simulink model "SIM_SAD_DEMO"  (R2025b)
settings: Solver=ode5  StartTime=0.0  StopTime=T/10  FixedStep=0.1  RelTol=1e-3
model workspace (MAT data in the model file):
  Pnull : Simulink.Parameter (value not decoded)
  rho_albedo_medio : Simulink.Parameter (value not decoded)
values from neighbouring files (symbols this model uses):
  Aree = zeros(10,1)    [SCRIPT_SAD_DEMO.m]    (also in lab_7.m)
  c = astroConstants(5)*1e3    [SCRIPT_SAD_DEMO.m]    (also in lab_7.m)
  draan = 1.99096871e-7    (= 1.99096871e-07)    [SCRIPT_SAD_DEMO.m]
  eps_E = deg2rad(astroConstants(63))    [SCRIPT_SAD_DEMO.m]    (also in lab_7.m)
  F_e = 1358    [SCRIPT_SAD_DEMO.m]    (also in lab_7.m)
  j_B = [0.01; 0.05; 0.01]    [SCRIPT_SAD_DEMO.m]    (also in lab_7.m)
  J_depl = [100.9, 0, 0;           0, 25.1, 0;           0, 0, 91.6]*1e-2    [SCRIPT_SAD_DEMO.m]    (also in lab_7.m)
  JD0 = juliandate(startTime)    [SCRIPT_SAD_DEMO.m]
  kep = [a,e,incl,raan,w,theta]    [SCRIPT_SAD_DEMO.m]    (also in lab_7.m)
  mu = astroConstants(13)    [SCRIPT_SAD_DEMO.m]    (also in lab_7.m)
  n = sqrt( (mu/ (a)^3))    [SCRIPT_SAD_DEMO.m]    (also in lab_7.m = sqrt((mu/ ((a/1000)^3))))
  n_sun = 2*pi/T_sun    (= 1.99238499086e-07)    [SCRIPT_SAD_DEMO.m]    (also in lab_7.m)
  Nmat = [ ... (first row only)    [SCRIPT_SAD_DEMO.m]    (also in lab_7.m)
  r_sun = 1*AU    [SCRIPT_SAD_DEMO.m]    (also in lab_7.m = 1*ua)
  Re = astroConstants(23)    [SCRIPT_SAD_DEMO.m]    (also in lab_7.m)
  rf = [ ... (first row only)    [SCRIPT_SAD_DEMO.m]    (also in lab_7.m)
  rhod = 0.1*ones(10,1)    [SCRIPT_SAD_DEMO.m]    (also in lab_7.m)
  rhos = zeros(10,1)    [SCRIPT_SAD_DEMO.m]    (also in lab_7.m)
  theta = 0    [SCRIPT_SAD_DEMO.m]    (also in lab_7.m)
symbols that are objects in the model workspace (value not decoded): Pnull, rho_albedo_medio
undefined symbols (not defined in the file or in its folder): avec, bvec, DiscIntNeverNeededParam, dspblkCoreblockFVToolHelper, gcbh, Gyro, Magmeter, q, SRP, Sun_sensor
libraries: LIBRARY_SAD x37, matrix_library x28
(part 3 of 3)

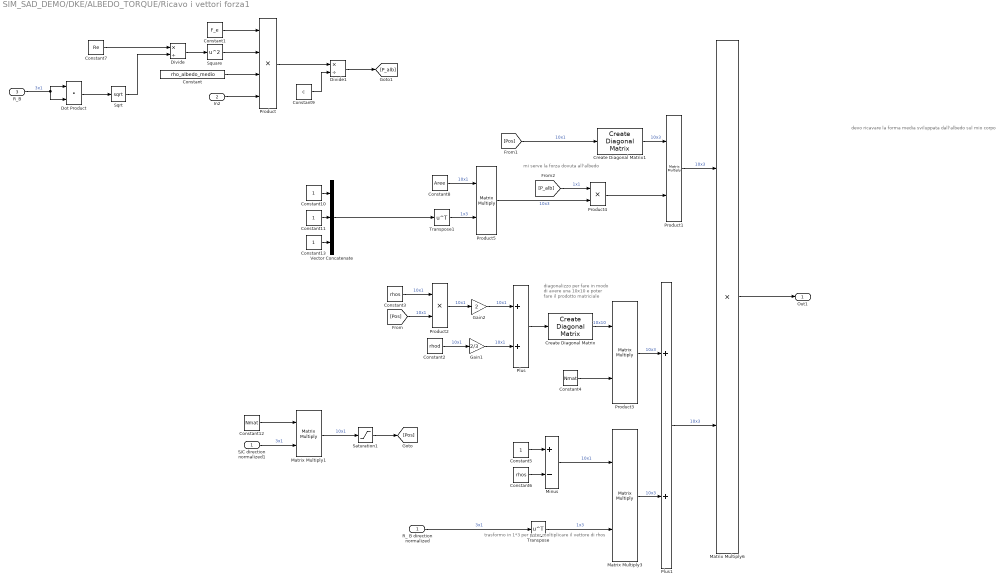
== system SIM_SAD_DEMO/DKE/ALBEDO_TORQUE/Ricavo i vettori forza1 ==
  note: devo ricavare la forma media sviluppata dall'albedo sul mio corpo
  note: mi serve la forza dovuta all'albedo
  note: diagonalizzo per fare in modo di avere una 10x10 e poter fare il prodotto matriciale
  note: trasformo in 1*3 per poter moltiplicare il vettore di rhos
  " R_ B direction normalized" : Inport
  In2 : Inport  Port=2
  R_B : Inport  Port=3
  Constant : Constant  Value=rho_albedo_medio
  Constant1 : Constant  Value=F_e
  Constant{5,10..11,13} (4 alike) : Constant
  Constant12 : Constant  Value=Nmat
  Constant2 : Constant  Value=rhod
  Constant3 : Constant  Value=rhos
  Constant4 : Constant  Value=Nmat
  Constant6 : Constant  Value=rhos
  Constant7 : Constant  Value=Re
  Constant8 : Constant  Value=Aree
  Constant9 : Constant  Value=c
  Create Diagonal Matrix : matrix_library/Create Diagonal Matrix
      settings: LibrarySourceBlock=|
      | simulink/Matrix
      | Operations/Create Diagonal
      | Matrix
  Create Diagonal Matrix1 : matrix_library/Create Diagonal Matrix
      settings: LibrarySourceBlock=|
      | simulink/Matrix
      | Operations/Create Diagonal
      | Matrix
  Divide : Product  Inputs=*/
  Divide1 : Product  Inputs=*/
  Dot Product : DotProduct  OutDataTypeStr=Inherit: Inherit via internal rule
  Gain1 : Gain  Gain=2/3
  Gain2 : Gain  Gain=2
  Matrix Multiply1 : Product  Multiplication=Matrix(*)
  Matrix Multiply3 : Product  Multiplication=Matrix(*)
  Matrix Multiply6 : Product
  Minus : Sum  Inputs=+-
  Plus : Sum
  Plus1 : Sum
  Product : Product  Inputs=4
  Product1 : Product  Multiplication=Matrix(*)
  Product2 : Product
  Product3 : Product  Multiplication=Matrix(*)
  Product4 : Product
  Product5 : Product  Multiplication=Matrix(*)
  S/C direction normalized1 : InportShadow
  Saturation1 : Saturate  UpperLimit=inf  LowerLimit=0
  Sqrt : Sqrt
  Square : Math  Operator=square
  Transpose : Math  Operator=transpose
  Transpose1 : Math  Operator=transpose
  Vector Concatenate : Concatenate  NumInputs=3
  Out1 : Outport
  wires:
  Gain1/1 -> Plus/2  "10x1"
  Plus1/1 -> Matrix Multiply6/2  "10x3"
  Product3/1 -> Plus1/1  "10x3"
  Constant4/1 -> Product3/2
  Product2/1 -> Gain2/1  "10x1"
  Constant2/1 -> Gain1/1  "10x1"
  Constant6/1 -> Minus/2
  Constant3/1 -> Product2/1  "10x1"
  Product1/1 -> Matrix Multiply6/1  "10x3"
  Gain2/1 -> Plus/1  "10x1"
  " R_ B direction normalized"/1 -> Transpose/1  "3x1"
  Matrix Multiply3/1 -> Plus1/2  "10x3"
  Constant5/1 -> Minus/1
  Matrix Multiply6/1 -> Out1/1
  [Pos] -> Create Diagonal Matrix1/1  "10x1"
  Matrix Multiply1/1 -> Saturation1/1  "10x1"
  Constant12/1 -> Matrix Multiply1/1
  Minus/1 -> Matrix Multiply3/1  "10x1"
  Transpose/1 -> Matrix Multiply3/2  "1x3"
  Saturation1/1 -> [Pos]
  [Pos] -> Product2/2  "10x1"
  Plus/1 -> Create Diagonal Matrix/1
  Constant13/1 -> Vector Concatenate/3
  Constant10/1 -> Vector Concatenate/1
  Constant11/1 -> Vector Concatenate/2
  Vector Concatenate/1 -> Transpose1/1
  Create Diagonal Matrix/1 -> Product3/1  "10x10"
  Transpose1/1 -> Product5/2  "1x3"
  Constant8/1 -> Product5/1  "10x1"
  Product5/1 -> Product4/2  "10x3"
  Create Diagonal Matrix1/1 -> Product1/1  "10x3"
  Product4/1 -> Product1/2
  S/C direction normalized1/1 -> Matrix Multiply1/2  "3x1"
  Constant7/1 -> Divide/1
  Divide/1 -> Square/1
  Constant1/1 -> Product/1
  Square/1 -> Product/2
  Constant/1 -> Product/3
  In2/1 -> Product/4
  Product/1 -> Divide1/1
  Constant9/1 -> Divide1/2
  Divide1/1 -> [P_alb]
  [P_alb] -> Product4/1  "1x1"
  Sqrt/1 -> Divide/2
  R_B/1 -> Dot Product/1, Dot Product/2  "3x1"
  Dot Product/1 -> Sqrt/1

== system SIM_SAD_DEMO/DKE/Earth radiation torque/Body 1 ==
  Constant : Constant  Value=SRP.body1.A
  Constant1 : Constant  Value=SRP.body1.N_hat
  Constant2 : Constant  Value=SRP.body1.rho_s
  Constant3 : Constant  Value=SRP.body1.rho_d
  A_i : Outport
  N_B_hat_i : Outport  Port=2
  rho_s_i : Outport  Port=3
  rho_d_i : Outport  Port=4
  wires:
  Constant/1 -> A_i/1
  Constant1/1 -> N_B_hat_i/1
  Constant2/1 -> rho_s_i/1
  Constant3/1 -> rho_d_i/1

== system SIM_SAD_DEMO/DKE/Earth radiation torque/Body 2 ==
  Constant : Constant  Value=SRP.body2.A
  Constant1 : Constant  Value=SRP.body2.N_hat
  Constant2 : Constant  Value=SRP.body2.rho_s
  Constant3 : Constant  Value=SRP.body2.rho_d
  A_i : Outport
  N_B_hat_i : Outport  Port=2
  rho_s_i : Outport  Port=3
  rho_d_i : Outport  Port=4
  wires:
  Constant3/1 -> rho_d_i/1
  Constant2/1 -> rho_s_i/1
  Constant1/1 -> N_B_hat_i/1
  Constant/1 -> A_i/1

== system SIM_SAD_DEMO/DKE/Earth radiation torque/Body 3 ==
  Constant : Constant  Value=SRP.body3.A
  Constant1 : Constant  Value=SRP.body3.N_hat
  Constant2 : Constant  Value=SRP.body3.rho_s
  Constant3 : Constant  Value=SRP.body3.rho_d
  A_i : Outport
  N_B_hat_i : Outport  Port=2
  rho_s_i : Outport  Port=3
  rho_d_i : Outport  Port=4
  wires:
  Constant/1 -> A_i/1
  Constant1/1 -> N_B_hat_i/1
  Constant2/1 -> rho_s_i/1
  Constant3/1 -> rho_d_i/1

== system SIM_SAD_DEMO/DKE/Earth radiation torque/Body 4 ==
  Constant : Constant  Value=SRP.body4.A
  Constant1 : Constant  Value=SRP.body4.N_hat
  Constant2 : Constant  Value=SRP.body4.rho_s
  Constant3 : Constant  Value=SRP.body4.rho_d
  A_i : Outport
  N_B_hat_i : Outport  Port=2
  rho_s_i : Outport  Port=3
  rho_d_i : Outport  Port=4
  wires:
  Constant3/1 -> rho_d_i/1
  Constant2/1 -> rho_s_i/1
  Constant1/1 -> N_B_hat_i/1
  Constant/1 -> A_i/1

== system SIM_SAD_DEMO/DKE/Earth radiation torque/Body 5 ==
  Constant : Constant  Value=SRP.body5.A
  Constant1 : Constant  Value=SRP.body5.N_hat
  Constant2 : Constant  Value=SRP.body5.rho_s
  Constant3 : Constant  Value=SRP.body5.rho_d
  A_i : Outport
  N_B_hat_i : Outport  Port=2
  rho_s_i : Outport  Port=3
  rho_d_i : Outport  Port=4
  wires:
  Constant/1 -> A_i/1
  Constant1/1 -> N_B_hat_i/1
  Constant2/1 -> rho_s_i/1
  Constant3/1 -> rho_d_i/1

== system SIM_SAD_DEMO/DKE/Earth radiation torque/Body 6 ==
  Constant : Constant  Value=SRP.body6.A
  Constant1 : Constant  Value=SRP.body6.N_hat
  Constant2 : Constant  Value=SRP.body6.rho_s
  Constant3 : Constant  Value=SRP.body6.rho_d
  A_i : Outport
  N_B_hat_i : Outport  Port=2
  rho_s_i : Outport  Port=3
  rho_d_i : Outport  Port=4
  wires:
  Constant3/1 -> rho_d_i/1
  Constant2/1 -> rho_s_i/1
  Constant1/1 -> N_B_hat_i/1
  Constant/1 -> A_i/1

== system SIM_SAD_DEMO/DKE/Earth radiation torque/Panel 1 ==
  Constant : Constant  Value=SRP.panel1.A
  Constant1 : Constant  Value=SRP.panel1.N_hat
  Constant2 : Constant  Value=SRP.panel1.rho_s
  Constant3 : Constant  Value=SRP.panel1.rho_d
  A_i : Outport
  N_B_hat_i : Outport  Port=2
  rho_s_i : Outport  Port=3
  rho_d_i : Outport  Port=4
  wires:
  Constant/1 -> A_i/1
  Constant1/1 -> N_B_hat_i/1
  Constant2/1 -> rho_s_i/1
  Constant3/1 -> rho_d_i/1

== system SIM_SAD_DEMO/DKE/Earth radiation torque/Panel 2 ==
  Constant : Constant  Value=SRP.panel2.A
  Constant1 : Constant  Value=SRP.panel2.N_hat
  Constant2 : Constant  Value=SRP.panel2.rho_s
  Constant3 : Constant  Value=SRP.panel2.rho_d
  A_i : Outport
  N_B_hat_i : Outport  Port=2
  rho_s_i : Outport  Port=3
  rho_d_i : Outport  Port=4
  wires:
  Constant3/1 -> rho_d_i/1
  Constant2/1 -> rho_s_i/1
  Constant1/1 -> N_B_hat_i/1
  Constant/1 -> A_i/1

== system SIM_SAD_DEMO/DKE/Earth radiation torque/Panel 3 ==
  Constant : Constant  Value=SRP.panel3.A
  Constant1 : Constant  Value=SRP.panel3.N_hat
  Constant2 : Constant  Value=SRP.panel3.rho_s
  Constant3 : Constant  Value=SRP.panel3.rho_d
  A_i : Outport
  N_B_hat_i : Outport  Port=2
  rho_s_i : Outport  Port=3
  rho_d_i : Outport  Port=4
  wires:
  Constant/1 -> A_i/1
  Constant1/1 -> N_B_hat_i/1
  Constant2/1 -> rho_s_i/1
  Constant3/1 -> rho_d_i/1

== system SIM_SAD_DEMO/DKE/Earth radiation torque/Panel 4 ==
  Constant : Constant  Value=SRP.panel4.A
  Constant1 : Constant  Value=SRP.panel4.N_hat
  Constant2 : Constant  Value=SRP.panel4.rho_s
  Constant3 : Constant  Value=SRP.panel4.rho_d
  A_i : Outport
  N_B_hat_i : Outport  Port=2
  rho_s_i : Outport  Port=3
  rho_d_i : Outport  Port=4
  wires:
  Constant3/1 -> rho_d_i/1
  Constant2/1 -> rho_s_i/1
  Constant1/1 -> N_B_hat_i/1
  Constant/1 -> A_i/1

== system SIM_SAD_DEMO/DKE/Earth-S//C Orbit/Conic Equation ==
  a : Inport
  e : Inport  Port=2
  theta_rad(t) : Inport  Port=3
  Constant : Constant  Value=2
  Constant1 : Constant
  Constant2 : Constant
  Cos : Trigonometry  Operator=cos
  Divide : Product  Inputs=*/
  Power : Math  Operator=pow
  Product : Product
  Product1 : Product
  Sum : Sum  Inputs=+-
  Sum1 : Sum
  r : Outport
  wires:
  a/1 -> Product/1
  e/1 -> Product1/1, Power/1
  Constant/1 -> Power/2
  Power/1 -> Sum/2
  Constant1/1 -> Sum/1
  Sum/1 -> Product/2
  Product/1 -> Divide/1
  Divide/1 -> r/1
  Constant2/1 -> Sum1/1
  theta_rad(t)/1 -> Cos/1
  Cos/1 -> Product1/2
  Product1/1 -> Sum1/2
  Sum1/1 -> Divide/2

== system SIM_SAD_DEMO/DKE/Earth-S//C Orbit/r (Inertial Frame) ==
  r : Inport
  theta_rad(t) : Inport  Port=2
  incl_rad : Inport  Port=3
  raan_rad : Inport  Port=4
  w_rad : Inport  Port=5
  Cos{,1..5} (6 alike) : Trigonometry  Operator=cos
  Product{,1,3,5} (4 alike) : Product
  Product2 : Product  Inputs=3
  Product4 : Product  Inputs=3
  Sin{,1..5} (6 alike) : Trigonometry
  Sum : Sum
  Sum1 : Sum  Inputs=+-
  Sum2 : Sum
  Vector Concatenate : Concatenate  NumInputs=3
  r_N : Outport
  wires:
  r/1 -> Product/1
  raan_rad/1 -> Cos/1, Cos4/1, Sin2/1, Sin/1
  w_rad/1 -> Sum/2
  Cos/1 -> Product1/2
  theta_rad(t)/1 -> Sum/1
  Sum/1 -> Sin4/1, Sin3/1, Cos3/1, Sin1/1, Cos1/1  "w+theta"
  Cos1/1 -> Product1/1
  Product1/1 -> Sum1/1
  Product2/1 -> Sum1/2
  Sin/1 -> Product2/1
  Sin1/1 -> Product2/2
  Cos2/1 -> Product2/3
  incl_rad/1 -> Cos5/1, Sin5/1, Cos2/1
  Sum1/1 -> Vector Concatenate/1
  Sum2/1 -> Vector Concatenate/2
  Sin2/1 -> Product3/1
  Cos3/1 -> Product3/2
  Product3/1 -> Sum2/1
  Product4/1 -> Sum2/2
  Cos4/1 -> Product4/1
  Sin3/1 -> Product4/2
  Cos5/1 -> Product4/3
  Sin4/1 -> Product5/1
  Sin5/1 -> Product5/2
  Product5/1 -> Vector Concatenate/3
  Vector Concatenate/1 -> Product/2
  Product/1 -> r_N/1

== system SIM_SAD_DEMO/DKE/Magnetic Torque/IGRF magnetic torque ==
  r_S/C_N : Inport
  Add : Sum  Inputs=+-
  Clock : Clock
  Constant : Constant  Value=JD0
  Constant2 : Constant  Value=Re
  Display{,1..3} (4 alike) : Display
  Gain : Gain  Gain=1000
  Gain1 : Gain  Gain=1000
  International Geomagnetic Reference Field : IGRF  time_in=off  month=January  day=1
      settings: AttributesFormatString=%<generation>
  MATLAB Function : MATLAB Function  TreatAsAtomicUnit=on
  MATLAB Function1 : MATLAB Function  TreatAsAtomicUnit=on
  MATLAB Function2 : MATLAB Function  TreatAsAtomicUnit=on
  MATLAB Function3 : LIBRARY_SAD/B_N (IGRF Model - Order N)/MATLAB Function3  SystemSampleTime=-1  VariantActivationTime=update diagram  EmptyChoice=off  PassThrough=off  PassThroughVariantControl=(default)  EmptyChoiceVariantControl=(default)  AllowFlexibleInterface=on  Latency=0  AutoFrameSizeCalculation=off
  Norm : Subsystem
  Scope : Scope
      settings: ActiveDisplayYMinimum=-1  ActiveDisplayYMaximum=1  DataLoggingVariableName=ScopeData23
  Scope1 : Scope
      settings: ActiveDisplayYMinimum=-1  ActiveDisplayYMaximum=1  DataLoggingVariableName=ScopeData24
  B_ECI : Outport
  wires:
  International Geomagnetic Reference Field/1 -> Scope1/1, MATLAB Function2/1(B_NED)
  MATLAB Function2/1(B_ECI) -> B_ECI/1
  Add/1 -> International Geomagnetic Reference Field/1, Display1/1
  Gain1/1 -> Add/1
  Clock/1 -> MATLAB Function/2(t), MATLAB Function2/4(t)
  MATLAB Function/1(r_ecef) -> MATLAB Function1/1(r_ecef)
  MATLAB Function1/1(lat) -> MATLAB Function2/2(lat_deg), Display2/1, International Geomagnetic Reference Field/2, Scope/1
  Gain/1 -> Add/2
  MATLAB Function1/2(lon) -> International Geomagnetic Reference Field/3, MATLAB Function2/3(lon_deg), Display3/1
  r_S/C_N/1 -> Norm/1(In1), MATLAB Function/1(r_eci)  "r_S/C_N"
  Constant/1 -> MATLAB Function3/1
  Norm/1(Out1) -> Gain1/1
  Constant2/1 -> Gain/1
  MATLAB Function3/1 -> MATLAB Function/3(alpha_G0), MATLAB Function2/5(alpha_G0), Display/1

== system SIM_SAD_DEMO/DKE/Solar Radiation Torque (SRP)/Body 1 ==
  Constant : Constant  Value=SRP.body1.A
  Constant1 : Constant  Value=SRP.body1.N_hat
  Constant2 : Constant  Value=SRP.body1.rho_s
  Constant3 : Constant  Value=SRP.body1.rho_d
  A_i : Outport
  N_B_hat_i : Outport  Port=2
  rho_s_i : Outport  Port=3
  rho_d_i : Outport  Port=4
  wires:
  Constant/1 -> A_i/1
  Constant1/1 -> N_B_hat_i/1
  Constant2/1 -> rho_s_i/1
  Constant3/1 -> rho_d_i/1

== system SIM_SAD_DEMO/DKE/Solar Radiation Torque (SRP)/Body 2 ==
  Constant : Constant  Value=SRP.body2.A
  Constant1 : Constant  Value=SRP.body2.N_hat
  Constant2 : Constant  Value=SRP.body2.rho_s
  Constant3 : Constant  Value=SRP.body2.rho_d
  A_i : Outport
  N_B_hat_i : Outport  Port=2
  rho_s_i : Outport  Port=3
  rho_d_i : Outport  Port=4
  wires:
  Constant3/1 -> rho_d_i/1
  Constant2/1 -> rho_s_i/1
  Constant1/1 -> N_B_hat_i/1
  Constant/1 -> A_i/1

== system SIM_SAD_DEMO/DKE/Solar Radiation Torque (SRP)/Body 3 ==
  Constant : Constant  Value=SRP.body3.A
  Constant1 : Constant  Value=SRP.body3.N_hat
  Constant2 : Constant  Value=SRP.body3.rho_s
  Constant3 : Constant  Value=SRP.body3.rho_d
  A_i : Outport
  N_B_hat_i : Outport  Port=2
  rho_s_i : Outport  Port=3
  rho_d_i : Outport  Port=4
  wires:
  Constant/1 -> A_i/1
  Constant1/1 -> N_B_hat_i/1
  Constant2/1 -> rho_s_i/1
  Constant3/1 -> rho_d_i/1

== system SIM_SAD_DEMO/DKE/Solar Radiation Torque (SRP)/Body 4 ==
  Constant : Constant  Value=SRP.body4.A
  Constant1 : Constant  Value=SRP.body4.N_hat
  Constant2 : Constant  Value=SRP.body4.rho_s
  Constant3 : Constant  Value=SRP.body4.rho_d
  A_i : Outport
  N_B_hat_i : Outport  Port=2
  rho_s_i : Outport  Port=3
  rho_d_i : Outport  Port=4
  wires:
  Constant3/1 -> rho_d_i/1
  Constant2/1 -> rho_s_i/1
  Constant1/1 -> N_B_hat_i/1
  Constant/1 -> A_i/1

== system SIM_SAD_DEMO/DKE/Solar Radiation Torque (SRP)/Body 5 ==
  Constant : Constant  Value=SRP.body5.A
  Constant1 : Constant  Value=SRP.body5.N_hat
  Constant2 : Constant  Value=SRP.body5.rho_s
  Constant3 : Constant  Value=SRP.body5.rho_d
  A_i : Outport
  N_B_hat_i : Outport  Port=2
  rho_s_i : Outport  Port=3
  rho_d_i : Outport  Port=4
  wires:
  Constant/1 -> A_i/1
  Constant1/1 -> N_B_hat_i/1
  Constant2/1 -> rho_s_i/1
  Constant3/1 -> rho_d_i/1

== system SIM_SAD_DEMO/DKE/Solar Radiation Torque (SRP)/Body 6 ==
  Constant : Constant  Value=SRP.body6.A
  Constant1 : Constant  Value=SRP.body6.N_hat
  Constant2 : Constant  Value=SRP.body6.rho_s
  Constant3 : Constant  Value=SRP.body6.rho_d
  A_i : Outport
  N_B_hat_i : Outport  Port=2
  rho_s_i : Outport  Port=3
  rho_d_i : Outport  Port=4
  wires:
  Constant3/1 -> rho_d_i/1
  Constant2/1 -> rho_s_i/1
  Constant1/1 -> N_B_hat_i/1
  Constant/1 -> A_i/1

== system SIM_SAD_DEMO/DKE/Solar Radiation Torque (SRP)/Panel 1 ==
  Constant : Constant  Value=SRP.panel1.A
  Constant1 : Constant  Value=SRP.panel1.N_hat
  Constant2 : Constant  Value=SRP.panel1.rho_s
  Constant3 : Constant  Value=SRP.panel1.rho_d
  A_i : Outport
  N_B_hat_i : Outport  Port=2
  rho_s_i : Outport  Port=3
  rho_d_i : Outport  Port=4
  wires:
  Constant/1 -> A_i/1
  Constant1/1 -> N_B_hat_i/1
  Constant2/1 -> rho_s_i/1
  Constant3/1 -> rho_d_i/1

== system SIM_SAD_DEMO/DKE/Solar Radiation Torque (SRP)/Panel 2 ==
  Constant : Constant  Value=SRP.panel2.A
  Constant1 : Constant  Value=SRP.panel2.N_hat
  Constant2 : Constant  Value=SRP.panel2.rho_s
  Constant3 : Constant  Value=SRP.panel2.rho_d
  A_i : Outport
  N_B_hat_i : Outport  Port=2
  rho_s_i : Outport  Port=3
  rho_d_i : Outport  Port=4
  wires:
  Constant3/1 -> rho_d_i/1
  Constant2/1 -> rho_s_i/1
  Constant1/1 -> N_B_hat_i/1
  Constant/1 -> A_i/1

== system SIM_SAD_DEMO/DKE/Solar Radiation Torque (SRP)/Panel 3 ==
  Constant : Constant  Value=SRP.panel3.A
  Constant1 : Constant  Value=SRP.panel3.N_hat
  Constant2 : Constant  Value=SRP.panel3.rho_s
  Constant3 : Constant  Value=SRP.panel3.rho_d
  A_i : Outport
  N_B_hat_i : Outport  Port=2
  rho_s_i : Outport  Port=3
  rho_d_i : Outport  Port=4
  wires:
  Constant/1 -> A_i/1
  Constant1/1 -> N_B_hat_i/1
  Constant2/1 -> rho_s_i/1
  Constant3/1 -> rho_d_i/1

== system SIM_SAD_DEMO/DKE/Solar Radiation Torque (SRP)/Panel 4 ==
  Constant : Constant  Value=SRP.panel4.A
  Constant1 : Constant  Value=SRP.panel4.N_hat
  Constant2 : Constant  Value=SRP.panel4.rho_s
  Constant3 : Constant  Value=SRP.panel4.rho_d
  A_i : Outport
  N_B_hat_i : Outport  Port=2
  rho_s_i : Outport  Port=3
  rho_d_i : Outport  Port=4
  wires:
  Constant3/1 -> rho_d_i/1
  Constant2/1 -> rho_s_i/1
  Constant1/1 -> N_B_hat_i/1
  Constant/1 -> A_i/1

== system SIM_SAD_DEMO/DKE/Magnetic Torque/IGRF magnetic torque/Norm ==
  note: square
  In1 : Inport
  Sqrt : Sqrt
  Square1 : Math  Operator=square
  Sum of Elements : Sum  Inputs=+
  Out1 : Outport
  wires:
  Square1/1 -> Sum of Elements/1
  Sqrt/1 -> Out1/1
  In1/1 -> Square1/1
  Sum of Elements/1 -> Sqrt/1

== matlab function SIM_SAD_DEMO/DKE/Magnetic Torque/IGRF magnetic torque/MATLAB Function ==
  data: r_eci input; r_ecef output; t input; alpha_G0 input
function r_ecef = eci2ecef(r_eci, t, alpha_G0)
% r_eci: [x, y, z] in meters (ECI frame)
% t: simulation time in seconds
% Default reference date: 1 Jan 2025 at 00:00 UTC

% Earth rotation rate (rad/s)
omega_earth = 7.2921159e-5;

% Compute Earth rotation angle
theta = alpha_G0 + omega_earth * t; % radians since reference epoch

% Rotation matrix about Z-axis
Rz = [cos(theta) sin(theta) 0;
     -sin(theta) cos(theta) 0;
      0          0          1];

% Convert ECI to ECEF
r_ecef = Rz * r_eci(:);
end

== matlab function SIM_SAD_DEMO/ATTITUDE DETERMINATION (q-method)/MATLAB Function ==
  data: u input; q output
function q = fcn(u)
% u: matrice K del q-method
% q: quaternione "continuo" (ambiguità di segno risolta)

persistent q_prev   % memorizza il quaternione del passo precedente

% 1) autovettore corrispondente all'autovalore massimo
[qvec, D] = eig(u);
[~, n] = max(real(diag(D)));
q = real(qvec(:, n));

% 2) normalizzo
q = q ./ norm(q);

% 3) se è la prima chiamata, non posso confrontare col passato
if isempty(q_prev)
    q_prev = q;
    return;
end

% 4) prodotto scalare col quaternione precedente
val = dot(q, q_prev);

% 5) se cambia ramo, flippa il segno
if val < 0
    q = -q;
end

% 6) aggiorna memoria
q_prev = q;
end

== matlab function SIM_SAD_DEMO/DKE/Magnetic Torque/IGRF magnetic torque/MATLAB Function1 ==
  data: r_ecef input; lat output; lon output
function [lat, lon] = ecef2latlon(r_ecef)
    x = r_ecef(1); y = r_ecef(2); z = r_ecef(3);
    lon = atan2(y, x);
    lat = atan2(z, sqrt(x^2 + y^2));
    lat = rad2deg(lat);
    lon = rad2deg(lon);
end

== matlab function SIM_SAD_DEMO/DKE/Magnetic Torque/IGRF magnetic torque/MATLAB Function2 ==
  data: B_NED input; B_ECI output; lat_deg input; lon_deg input; t input; alpha_G0 input
function B_ECI = ned2eci(B_NED, lat_deg, lon_deg, t,alpha_G0)
    % Converts magnetic field from NED frame to ECI frame
    % Inputs:
    %   B_NED   : [Bx, By, Bz] in NED frame (Tesla or Gauss)
    %   lat_deg : latitude in degrees
    %   lon_deg : longitude in degrees
    %   t       : simulation time in seconds (since reference epoch)
    %
    % Output:
    %   B_ECI   : magnetic field in ECI frame
    
    % Convert degrees to radians
    lat = deg2rad(lat_deg);
    lon = deg2rad(lon_deg);
    
    % Earth rotation rate (rad/s)
    omega_earth = 7.2921159e-5;
    
    % Earth rotation angle since reference epoch (1 Jan 2025)
    theta = alpha_G0 + omega_earth * t;
    
    % --- Step 1: NED → ECEF rotation matrix ---
    R_NED2ECEF = [-sin(lat)*cos(lon), -sin(lon),  -cos(lat)*cos(lon);
                  -sin(lat)*sin(lon), cos(lon),   -cos(lat)*sin(lon);
                  cos(lat),             0,        -sin(lat)];
    
    % Convert B_NED to ECEF
    B_ECEF = R_NED2ECEF * B_NED(:);
    
    % --- Step 2: ECEF → ECI rotation matrix ---
    R_ECEF2ECI = [cos(theta), -sin(theta), 0;
                  sin(theta),  cos(theta), 0;
                  0,           0,          1];
    
    % Convert B_ECEF to ECI
    B_ECI = R_ECEF2ECI * B_ECEF * 1e-9;
end
